simulink model "TEST_TCP"  (R2022b)
settings: Solver=FixedStepAuto  StartTime=0.0  StopTime=inf  FixedStep=1e-3  RelTol=1e-3  EnableMultiTasking=on
undefined symbols (not defined in the file or in its folder): angular, CIRCUIT, CLTF_DAMP, CLTF_FREQ, CLTF_GAIN, CONTROL, CONTROL_INI, DiscIntNeverNeededParam, INPUT, linear, MCP3201, MD25, MODEL, MODEL_INI, mpcstate, MPU60X0, MPU9250, MSG, NAV_MPC_CONTROL, OUTPUT, RCRX, SAMPLING_TIME, SYSID_INPUT, VL6180X
libraries: raspberrypiCommlib x156, simulink x86, dspsigattribs x14, raspberrypiNetworklib x13, embedlinuxBasiclib x9, ctrlSharedLib x2, ros2lib x2, mpclib x1, vrlib x1, sldrtlib x1
(part 17 of 17)

== matlab function TEST_TCP/CONTROL/LOCAL TARGETS/NAVIGATION TARGETS/TRAJECTORY PLANNER (POLYNOMIAL IN Vx & Vy) ==
  data: CONTROL_IN input Bus: CONTROL_Bus; CONTROL output Bus: CONTROL_Bus
function CONTROL = MPC_TARGET_UPDATE(CONTROL_IN)

%--------------------------------------------------------------
% COPY CONTROL BUS
%--------------------------------------------------------------
CONTROL = CONTROL_IN;

%--------------------------------------------------------------
% DISABLING TARGET UPDATE
%--------------------------------------------------------------
% CONTROL_STATUS
% / 0. INITIALIZATION     / 1. ESTIMATION    / 2. ACTIVE CONTROL
if CONTROL.STATE.CONTROL_STATUS < 2  % INITIALIZATION    
    return
end

%--------------------------------------------------------------
% TIME MANAGEMENT
%--------------------------------------------------------------
% Sampling time 
ts = CONTROL.PARAM.SAMPLING_TIME;
% Trajectory update time 
tc = 10*ts;
persistent initialize TIMER
if isempty(initialize)
    TIMER = 0;
    initialize = 1;
end
TIMER = TIMER + ts;
if TIMER > tc-ts/2
    TIMER = 0;
    return
end

%--------------------------------------------------------------
% PARAMETERS
%--------------------------------------------------------------
% Maximun velocity magnitude 
VEL_MAG_MAX = CONTROL.PARAM.VEL_MAG_MAX;
% Prediction horizon (<= prediction horizon in mpcDesigner)
P = 20;
% Circular outline radius
% WP_R = CONTROL.PARAM.WP_R;

%--------------------------------------------------------------
% MEASUREMENTS AND STATE
%--------------------------------------------------------------
VEL_MAG = CONTROL.INPUT.FORWARD_VEL;
VEL_ANG = CONTROL.INPUT.YAW_ANG;
VEL_X = CONTROL.INPUT.EARTH_VEL(1);
VEL_Y = CONTROL.INPUT.EARTH_VEL(2);
POS_XY = CONTROL.INPUT.EARTH_POS(1:2);
WP_XY = CONTROL.TARGET.MISSION_WAYPOINTS(1:CONTROL.TARGET.MISSION_NUM_WAYPOINTS,2:3)';
NEXT_WP = CONTROL.TARGET.MISSION_COUNT;
M = CONTROL.PARAM.NAV_MPC.PRED_HRZ;
if NEXT_WP == size(WP_XY,2)
    CONTROL.TARGET.NAV_REF_LC(1) = 0;
    CONTROL.TARGET.NAV_REF(1) = 0;
    CONTROL.TARGET.NAV_REF_MPC(1:M,1) = zeros(M,1);
    CONTROL.TARGET.VEL_XY_REF(1) = 0;
    CONTROL.TARGET.VEL_XY_REF(2) = 0;
    CONTROL.TARGET.FORWARD_VEL_REF = 0;
end

%--------------------------------------------------------------
% TRAJECTORY PLANNING
%--------------------------------------------------------------
% x(t) = sum(ai*t^i) i=0...N
% y(t) = sum(bi*t^i) i=0...N
% dx(t)/dt = vx(t) = sum(i*ai*t^(i-1)) i=0...N
% dy(t)/dt = vy(t) = sum(i*bi*t^(i-1)) i=0...N
% Position and distance data
pos_x = [POS_XY(1) WP_XY(1,NEXT_WP:end)]';
pos_y = [POS_XY(2) WP_XY(2,NEXT_WP:end)]'; 
d = abs(diff(pos_x) + 1j*diff(pos_y));
% Delete duplicated points (distance = 0)
ind = find(d>0);
pos_x = [pos_x(ind) ; pos_x(end)];
pos_y = [pos_y(ind) ; pos_y(end)];
d = abs(diff(pos_x) + 1j*diff(pos_y));
% Polynomial parameters
Np = min([4 length(pos_x)+1]);
% Polynomial order
N = Np-1;
% Parameter initialization
a = zeros(Np,1);
b = zeros(Np,1);
a(1) = pos_x(1);
b(1) = pos_y(1);
a(2) = VEL_X;
b(2) = VEL_Y;
% Time vector for target
t_tgt = (1:P)'*tc;
VEL_MAG_TARGET = zeros(P,1);
VEL_ANG_TARGET = zeros(P,1);
% Time matrix for velocity target computation
matTp = zeros(P,N+1);
matTv = zeros(P,N);
for nn = 1:N+1
    matTp(:,nn) = t_tgt.^(nn-1);
end
for nn = 1:N
    matTv(:,nn) = nn*t_tgt.^(nn-1);
end
flag_vel_max = true;
k = 1;
while flag_vel_max
    % Reaching time for the next waypoints
    t = cumsum([0 ; k*sqrt(2)*d(1:N-1)/VEL_MAG_MAX]);    
    % Polynomial coefficient estimation 
    % matBx = matA*a(3:Np);  
    % matBy = matA*b(3:Np)
    matA = zeros(Np-2);
    for nn = 1:Np-2
        matA(:,nn) = t(2:end).^(nn+1);
    end
    matBx = pos_x(2:Np-1) - a(2)*t(2:end) - a(1);
    matBy = pos_y(2:Np-1) - b(2)*t(2:end) - b(1);
    inv_matA = inv(matA);
    a(3:end) = inv_matA*matBx;
    b(3:end) = inv_matA*matBy;
    % Position target calculation
    px_tgt = matTp*a;
    py_tgt = matTp*b; 
    % Magnitude and angle velocity targets calculation
    vx_tgt = matTv*a(2:end);
    vy_tgt = matTv*b(2:end); 
    v_tgt = vx_tgt + 1j*vy_tgt;
    VEL_MAG_TARGET = abs(v_tgt);
    VEL_ANG_TARGET = angle(v_tgt)*(VEL_MAG_TARGET(1)>=0.005) + ...
                    VEL_ANG*ones(size(VEL_ANG_TARGET))*(VEL_MAG_TARGET(1)<0.005);
    % Decreasing velocity factor
    k = k*max(VEL_MAG_TARGET)/VEL_MAG_MAX;
    % Maximun velocity verification
    if (max(VEL_MAG_TARGET)/VEL_MAG_MAX)<=1.01
        flag_vel_max = false;
    end
end

%--------------------------------------------------------------
% UNWRAPPING
%--------------------------------------------------------------
aux1 = VEL_ANG_TARGET(1);
aux2 = VEL_ANG;
INC_VEL_ANG_TARGET = zeros(21,1);
INC_VEL_ANG_TARGET(1) = aux1-aux2;
for nn=1:10
    INC_VEL_ANG_TARGET(2*nn:2*nn+1) = [aux1-aux2-2*nn*pi ; aux1-aux2+2*nn*pi];
end
[~,ind] = min(abs(INC_VEL_ANG_TARGET));
VEL_ANG_TARGET(1) = aux2 + INC_VEL_ANG_TARGET(ind);
for nn = 2:P
    INC_VEL_ANG_TARGET = [VEL_ANG_TARGET(nn)-VEL_ANG_TARGET(nn-1)
                          VEL_ANG_TARGET(nn)-VEL_ANG_TARGET(nn-1)-2*pi
                          VEL_ANG_TARGET(nn)-VEL_ANG_TARGET(nn-1)+2*pi];
    [~,ind] = min(abs(INC_VEL_ANG_TARGET));
    VEL_ANG_TARGET(nn) = VEL_ANG_TARGET(nn-1) + INC_VEL_ANG_TARGET(ind);
end

%--------------------------------------------------------------
% CONTROL BUS UPDATE
%--------------------------------------------------------------
CONTROL.TARGET.NAV_REF_LC(1) = VEL_MAG_TARGET(1);
CONTROL.TARGET.NAV_REF_LC(2) = VEL_ANG_TARGET(1);
if M<=P
    CONTROL.TARGET.NAV_REF_MPC(1:M,1) = VEL_MAG_TARGET(1:M);
    CONTROL.TARGET.NAV_REF_MPC(1:M,2) = VEL_ANG_TARGET(1:M);
else
    CONTROL.TARGET.NAV_REF_MPC(1:M,1) = [VEL_MAG_TARGET(1:P); VEL_MAG_TARGET(end)*ones(M-P,1)];
    CONTROL.TARGET.NAV_REF_MPC(1:M,2) = [VEL_ANG_TARGET(1:P); VEL_ANG_TARGET(end)*ones(M-P,1)];
end
VEL_XY = VEL_MAG_TARGET.*exp(1j*VEL_ANG_TARGET);
CONTROL.TARGET.VEL_XY_REF(1) = real(VEL_XY(1));
CONTROL.TARGET.VEL_XY_REF(2) = imag(VEL_XY(1));
CONTROL.TARGET.NAV_REF = [VEL_MAG_TARGET(1) ; VEL_ANG_TARGET(1)];

return

== matlab function TEST_TCP/CONTROL/CONTROL UPDATE  ==
  data: CONTROL_IN input Bus: CONTROL_Bus; CONTROL output Bus: CONTROL_Bus; MOTOR_VOLT output size=2; MOTOR_VOLT_CD output size=2
function [CONTROL,MOTOR_VOLT,MOTOR_VOLT_CD] = CONTROL_UPDATE(CONTROL_IN)

%--------------------------------------------------------------
% COPY CONTROL BUS
%--------------------------------------------------------------
CONTROL = CONTROL_IN;

%--------------------------------------------------------------
% TIMER FOR DIGITAL CONTROL SAMPLING TIME
%--------------------------------------------------------------
persistent TIMER init_1
if isempty(init_1)
    TIMER = 0;
    init_1 = 1;
end
TIMER = TIMER + CONTROL.PARAM.SAMPLING_TIME;

%--------------------------------------------------------------
% CONTROL STATUS
%--------------------------------------------------------------
% / 0. INITIALIZATION     / 1. ESTIMATION    / 2. ACTIVE CONTROL
CONTROL_STATUS = CONTROL.STATE.CONTROL_STATUS;
NUM_DLYS = uint8(floor(CONTROL.PARAM.MOTOR_DELAY/CONTROL.PARAM.CONTROL_SAMPLING_TIME));
if CONTROL_STATUS == 0 || CONTROL_STATUS == 1  % INITIALIZATION OR ESTIMATION
    MOTOR_VOLT = zeros(2,1);
    MOTOR_VOLT_CD = zeros(2,1);
    return
end 

%--------------------------------------------------------------
% DIGITAL CONTROL SAMPLING TIME MANAGEMENT
%--------------------------------------------------------------
if TIMER < CONTROL.PARAM.CONTROL_SAMPLING_TIME
    MOTOR_VOLT = CONTROL.OUTPUT.MOTOR_VOLT;
    MOTOR_VOLT_CD = CONTROL.OUTPUT.MOTOR_VOLT_CD;
    return
else
    TIMER = 0;
end

%--------------------------------------------------------------
% CONTROL MODE
%--------------------------------------------------------------
% / 0. OPEN LOOP / 1. ATTITUDE / 2. VELOCITY / 3. NAVIGATION / 
% / 4. WALL FOLLOWER / 5. WALL-FOLLOWER COMPETITION / 
% / 6. NAVIGATION COMPETITION / 7.FORWARD VELOCITY COMPETITION
CONTROL_MODE = CONTROL.STATE.CONTROL_MODE;
%--------------------------------------------------------------
% VEHICLE MODE
%--------------------------------------------------------------
% / 0. CAR / 1. SELF-BALANCING VEHICLE
VEHICLE_MODE = CONTROL.STATE.VEHICLE_MODE;

%--------------------------------------------------------------
% CONTROL STATE
%--------------------------------------------------------------
persistent init_2 PA_REF_PRV PA_MO_PRV PA_MV_PRV PA_MOD_PRV ...
                      PA_INT_PID_PRV PA_DER_PID_PRV ...
                      YA_REF_PRV YA_MO_PRV YA_MV_PRV YA_MOD_PRV ...
                      YA_INT_PID_PRV YA_DER_PID_PRV ...
                      YR_REF_PRV YR_MO_PRV YR_MV_PRV ...
                      YR_INT_PID_PRV YR_DER_PID_PRV  ...
                      FV_REF_PRV FV_MO_PRV FV_MV_PRV ...
                      FV_INT_PID_PRV FV_DER_PID_PRV  ...
                      WFL_REF_PRV WFL_MO_PRV WFL_MV_PRV ...
                      WFL_INT_PID_PRV WFL_DER_PID_PRV ...
                      SFC_REF_PRV SFC_MO_PRV SFC_MV_PRV ...
                      SFC_STATE_PRV SFC_STATE_INT_PRV  ...
                      NAV_STATE_PRV NAV_STATE_INT_PRV NAV_MV_PRV ...
                      NAV_MO_PRV NAV_REF_PRV ...
                      VEL_SP_STATE YAW_RATE_SP_STATE ...
                      FV_DB_ERR_PRV YR_DB_ERR_PRV FV_DB_MV_PRV YR_DB_MV_PRV ...
                      MAT_NAV_LQR_GS
                                       
% Size of vector and matrices
% Initialization
if isempty(init_2) || CONTROL.STATE.CURRENT_STATUS_SYS==11 % STOP
    PA_REF_PRV = 0;
    PA_MO_PRV = 0;
    PA_MV_PRV = 0;
    PA_MOD_PRV = 0;
    PA_INT_PID_PRV = 0;
    PA_DER_PID_PRV = 0;
    YA_REF_PRV = 0;
    YA_MO_PRV = 0;
    YA_MV_PRV = 0;
    YA_MOD_PRV = 0;
    YA_INT_PID_PRV = 0;
    YA_DER_PID_PRV = 0;
    YR_REF_PRV = 0;
    YR_MO_PRV = 0;
    YR_MV_PRV = 0;
    YR_INT_PID_PRV = 0;
    YR_DER_PID_PRV = 0;
    FV_REF_PRV = 0;
    FV_MO_PRV = 0;
    FV_MV_PRV = 0;
    FV_INT_PID_PRV = 0;
    FV_DER_PID_PRV = 0;
    WFL_REF_PRV = 0.1;
    WFL_MO_PRV = 0.1; 
    WFL_MV_PRV = 0;
    WFL_INT_PID_PRV = 0;
    WFL_DER_PID_PRV = 0;
    SFC_REF_PRV = zeros(2,1);
    SFC_MO_PRV = zeros(2,1);
    SFC_MV_PRV = zeros(2,2);
    SFC_STATE_INT_PRV = zeros(2,1);       
    SFC_STATE_PRV = zeros(6,1);
    SFC_STATE_PRV(4) = CONTROL.INPUT.WALL_DIST; 
    VEL_SP_STATE = zeros(NUM_DLYS+2,1);
    NAV_MV_PRV = zeros(2,2);       
    NAV_STATE_PRV = zeros(6,1);
    NAV_STATE_INT_PRV = zeros(2,1);
    NAV_MO_PRV = zeros(2,1);
    NAV_REF_PRV = zeros(2,1);
    YAW_RATE_SP_STATE = zeros(NUM_DLYS+2,1);
    FV_DB_ERR_PRV = zeros(1,2);
    YR_DB_ERR_PRV = zeros(1,2);
    FV_DB_MV_PRV = zeros(1,2);
    YR_DB_MV_PRV = zeros(1,2);  
    N_calphao = length(CONTROL.PARAM.NAV_SFC.COS_ANG);
    N_vo = length(CONTROL.PARAM.NAV_SFC.FV);
    N_invro = length(CONTROL.PARAM.NAV_SFC.INV_DIST);
    MAT_NAV_LQR_GS = zeros(N_calphao*N_vo*N_invro,3);
    calphao = CONTROL.PARAM.NAV_SFC.COS_ANG;
    vo = CONTROL.PARAM.NAV_SFC.FV;
    invro = CONTROL.PARAM.NAV_SFC.INV_DIST;
    nn = 0;
    for ii = 1:N_calphao
        for jj = 1:N_vo
            for kk = 1:N_invro
                nn = nn + 1;
                MAT_NAV_LQR_GS(nn,:) = [calphao(ii) vo(jj) invro(kk)];
            end
        end
    end
    init_2 = 1;
end

%--------------------------------------------------------------
% INITIALIZATION
%--------------------------------------------------------------
MOTOR_VOLT_CD = zeros(2,1);
NAV_TARGET_REACHED = false;

%-------------------------------------------------------------------------
% ADAPTIVE CONTROL: GAIN SCHEDULING
%-------------------------------------------------------------------------
if CONTROL.STATE.GAIN_SCHEDULING
    % Filtered scheduling variable
    SCHED_VAR = CONTROL.TARGET.FORWARD_VEL_REF;
    % Scheduling variables at operating points
    SCHED_OP = CONTROL.PARAM.OP_STATE(1,:);
    [~,NUM_OP] = min(abs(SCHED_OP-SCHED_VAR));
else
    NUM_OP = double(CONTROL.STATE.FORWARD_VEL_MAIN_OP);
end

%-------------------------------------------------------------------------
% NAVIGATION: ADAPTIVE LQR CONTROL (GAIN SCHEDULING)
%-------------------------------------------------------------------------
if (CONTROL_MODE==3 || CONTROL_MODE==6) && VEHICLE_MODE==0 && ...
              CONTROL.STATE.NAV_CONTROL_TYPE==0
    % OUTPUT COMPUTATION IN POLAR COORDINATES
    NAV_MO_XY = CONTROL.TARGET.NAV_REF - CONTROL.INPUT.NAV_MO;
    NAV_MO_MAG = norm(NAV_MO_XY); % r
    if CONTROL.STATE.NAV_TARGET_REACHED==0
        aux1 = atan2(NAV_MO_XY(2),NAV_MO_XY(1));
        aux2 = CONTROL.TARGET.YAW_ANG_REF;
        INC_ANG = zeros(41,1);
        INC_ANG(1) = aux1-aux2;
        for ii = 1:20
            INC_ANG(2*ii)   = aux1-aux2-2*ii*pi;
            INC_ANG(2*ii+1) = aux1-aux2+2*ii*pi;
        end
        [~,ind] = min(abs(INC_ANG));
        CONTROL.TARGET.YAW_ANG_REF = aux2 + INC_ANG(ind); % phi
    end
    NAV_MO_ANG = CONTROL.TARGET.YAW_ANG_REF - CONTROL.INPUT.YAW_ANG; % alpha = phi - shi
    if abs(NAV_MO_MAG)>CONTROL.PARAM.NAV_MAX_TARGET_RADIUS
        NAV_MO_MAG = CONTROL.PARAM.NAV_MAX_TARGET_RADIUS; % r
    end
    NAV_STATE = [CONTROL.INPUT.FORWARD_VEL ; CONTROL.INPUT.YAW_RATE ; ...
                 CONTROL.INPUT.FV_INT_ERROR ; CONTROL.INPUT.YR_INT_ERROR ; ...
                 NAV_MO_MAG ; NAV_MO_ANG];
    if NAV_MO_MAG<=CONTROL.PARAM.NAV_STOP_RADIUS
       NAV_MO_MAG = 0; % r = 0
       NAV_MO_ANG = 0; % alpha = 0;
       NAV_STATE = zeros(6,1);
       NAV_STATE_PRV = zeros(6,1);
       NAV_STATE_INT_PRV = zeros(2,1);
       NAV_MO_PRV = zeros(2,1);
       NAV_REF_PRV = zeros(2,1);
       CONTROL.STATE.NAV_TARGET_REACHED = uint8(1);
    else
        CONTROL.STATE.NAV_TARGET_REACHED = uint8(0);
    end
    NAV_REF = [0 ; 0];
    NAV_MO = [NAV_MO_MAG ; NAV_MO_ANG];
    % GAIN MATRICES TO BE APPLIED
    SANG = sin(NAV_MO_ANG);
    signSANG = SANG>=0;
    CANG = cos(NAV_MO_ANG);
    signCANG = CANG>=0;
    absCANG = abs(CANG);    
    FV = CONTROL.INPUT.FORWARD_VEL;
    INVR = (1/(NAV_MO_MAG+(NAV_MO_MAG<0.01)))*(NAV_MO_MAG>0.01) + 100*(NAV_MO_MAG<=0.01);
    if signCANG && signSANG
        NAV_MATRIX = CONTROL.PARAM.NAV_SFC.KPP;
    elseif signCANG && ~signSANG
        NAV_MATRIX = CONTROL.PARAM.NAV_SFC.KPN;
    elseif ~signCANG && signSANG
        NAV_MATRIX = CONTROL.PARAM.NAV_SFC.KNP;
    else
        NAV_MATRIX = CONTROL.PARAM.NAV_SFC.KNN;
    end
    [~,ind] = min(sum(abs([MAT_NAV_LQR_GS(:,1:2) MAT_NAV_LQR_GS(:,3)/100]-repmat([absCANG FV INVR/100],size(NAV_MATRIX,1),1)),2));
    % INPUTS
    NAV_INPUT.MO_PRV = NAV_MO_PRV;
    NAV_INPUT.REF_PRV = NAV_REF_PRV;
    NAV_INPUT.STATE_PRV = NAV_STATE_PRV;
    NAV_INPUT.STATE = NAV_STATE;
    NAV_INPUT.MV_PRV = NAV_MV_PRV;
    NAV_INPUT.STATE_INT = NAV_STATE_INT_PRV;
    % PARAMETERS
    NAV_PARAM.ts = CONTROL.PARAM.CONTROL_SAMPLING_TIME;
    NAV_PARAM.MV_MAX = CONTROL.PARAM.NAV_MV_MAX;
    NAV_PARAM.MV_MIN = CONTROL.PARAM.NAV_MV_MIN;
    NAV_PARAM.OP_INPUT = zeros(2,1);
    NAV_PARAM.OP_STATE = zeros(6,1);
    NAV_PARAM.OP_OUTPUT = zeros(2,1);
    NAV_PARAM.Kr = zeros(2,2);
    NAV_PARAM.Kd = zeros(2,2);
    NAV_PARAM.K = [NAV_MATRIX(ind,1:6) ; NAV_MATRIX(ind,7:12)];
    NAV_PARAM.Ki = [NAV_MATRIX(ind,13:14) ; NAV_MATRIX(ind,15:16)];
    NAV_PARAM.INT_DISC_TYPE = CONTROL.PARAM.FORWARD_VEL_SFC.INT_DISC_TYPE;
    NAV_PARAM.ANTIWINDUP = uint8(1);
    NAV_INPUT.REF = NAV_REF;
    NAV_INPUT.MO = NAV_MO;
    % STATE-FEEDBACK CONTROL
    NAV_OUTPUT = SFC(NAV_INPUT,NAV_PARAM);
    % OUTPUTS
    NAV_MV_PRV = [NAV_OUTPUT.MV NAV_MV_PRV(:,1:end-1)];
    NAV_REF_PRV = NAV_INPUT.REF;
    NAV_MO_PRV = NAV_INPUT.MO;
    NAV_STATE_PRV = NAV_INPUT.STATE;
    NAV_STATE_INT_PRV = NAV_OUTPUT.STATE_INT; 
    if CONTROL.STATE.NAV_TARGET_REACHED==0
        CONTROL.TARGET.FORWARD_VEL_REF = NAV_OUTPUT.MV(1);
        CONTROL.TARGET.YAW_RATE_REF = NAV_OUTPUT.MV(2);
    else
        CONTROL.TARGET.FORWARD_VEL_REF = 0;
        CONTROL.TARGET.YAW_RATE_REF = 0;
    end
end

%-------------------------------------------------------------------------
% WALL DISTANCE: PID 
%-------------------------------------------------------------------------
if (CONTROL_MODE==4 || CONTROL_MODE==5) && CONTROL.STATE.WFL_CONTROL_TYPE<2  
    % INPUTS
    PID_INPUT.REF = CONTROL.TARGET.WALL_DIST_REF;
    PID_INPUT.REF_PRV = WFL_REF_PRV;
    PID_INPUT.MO = CONTROL.INPUT.WALL_DIST;
    PID_INPUT.MO_PRV = WFL_MO_PRV;
    PID_INPUT.INT_PID_PRV = WFL_INT_PID_PRV;
    PID_INPUT.DER_PID_PRV = WFL_DER_PID_PRV;
    PID_INPUT.MV_PRV = WFL_MV_PRV(1);
    PID_INPUT.MOD = 0;
    PID_INPUT.MOD_PRV = 0;
    PID_INPUT.MV_PID_PRV = 0;
    PID_INPUT.STATE = 0;
    PID_INPUT.STATE_PRV = 0;
    PID_INPUT.STATE_DCP = 0;
    % PARAMETERS
    PID_PARAM.ts = CONTROL.PARAM.CONTROL_SAMPLING_TIME;
    if CONTROL.STATE.WFL_CONTROL_TYPE
        PID_PARAM.K = CONTROL.PARAM.WFL_CD_PID.K(NUM_OP,1);
        PID_PARAM.Ti = CONTROL.PARAM.WFL_CD_PID.Ti(NUM_OP,1);
        PID_PARAM.Td = CONTROL.PARAM.WFL_CD_PID.Td(NUM_OP,1);
        PID_PARAM.b = CONTROL.PARAM.WFL_CD_PID.b(NUM_OP,1);
        PID_PARAM.N = CONTROL.PARAM.WFL_CD_PID.N(NUM_OP,1);
        PID_PARAM.MV_MAX = 1e6;
        PID_PARAM.MV_MIN = -1e6;
        PID_PARAM.INT_DISC_TYPE = CONTROL.PARAM.WFL_CD_PID.INT_DISC_TYPE;
        PID_PARAM.DER_DISC_TYPE = CONTROL.PARAM.WFL_CD_PID.DER_DISC_TYPE;
        PID_PARAM.DER_INPUT = CONTROL.PARAM.WFL_CD_PID.DER_INPUT;
        PID_PARAM.ANTIWINDUP = CONTROL.PARAM.WFL_CD_PID.ANTIWINDUP;
    else
        PID_PARAM.K = CONTROL.PARAM.WFL_SL_PID.K(NUM_OP,1);
        PID_PARAM.Ti = CONTROL.PARAM.WFL_SL_PID.Ti(NUM_OP,1);
        PID_PARAM.Td = CONTROL.PARAM.WFL_SL_PID.Td(NUM_OP,1);
        PID_PARAM.b = CONTROL.PARAM.WFL_SL_PID.b(NUM_OP,1);
        PID_PARAM.N = CONTROL.PARAM.WFL_SL_PID.N(NUM_OP,1);
        PID_PARAM.MV_MAX = 1e6;
        PID_PARAM.MV_MIN = -1e6;
        PID_PARAM.INT_DISC_TYPE = CONTROL.PARAM.WFL_SL_PID.INT_DISC_TYPE;
        PID_PARAM.DER_DISC_TYPE = CONTROL.PARAM.WFL_SL_PID.DER_DISC_TYPE;
        PID_PARAM.DER_INPUT = CONTROL.PARAM.WFL_SL_PID.DER_INPUT;
        PID_PARAM.ANTIWINDUP = CONTROL.PARAM.WFL_SL_PID.ANTIWINDUP;
    end
    % PID CONTROL
    PID_OUTPUT = PID_MV(PID_INPUT,PID_PARAM);
    % OUTPUTS
    WFL_MV_PRV = PID_OUTPUT.MV;
    if CONTROL.STATE.WFL_CONTROL_TYPE
        CONTROL.TARGET.YAW_ANG_REF = PID_OUTPUT.MV;
    else
        MOTOR_VOLT_CD(2) = PID_OUTPUT.MV + ...
            double(CONTROL.STATE.WFL_FEEDFORWARD)*CONTROL.PARAM.MOTOR_VOLT_DROP_DIF;
    end
    WFL_REF_PRV = CONTROL.TARGET.WALL_DIST_REF;
    WFL_MO_PRV = CONTROL.INPUT.WALL_DIST;
    WFL_INT_PID_PRV = PID_OUTPUT.INT;
    WFL_DER_PID_PRV = PID_OUTPUT.DER;
end

%-------------------------------------------------------------------------
% STATE FEEDBACK CONTROL DEFINITION
%-------------------------------------------------------------------------
SFC_PARAM.K = zeros(2,6);
SFC_PARAM.Ki = zeros(2,2);
SFC_PARAM.Kr = zeros(2,2);
SFC_PARAM.Kd = zeros(2,2);
SFC_PARAM.INT_DISC_TYPE = uint8(0);
SFC_PARAM.ANTIWINDUP = uint8(0);
SFC_INPUT.REF = zeros(2,1);
SFC_INPUT.MO = zeros(2,1);
SFC_PARAM.OP_OUTPUT = zeros(2,1);
FLAG_SFC = uint8(0);
FLAG_MV = uint8([0 0]);
% FORWARD VELOCITY AND STATE FEEDBACK CONTROL AND CAR MODE
if CONTROL_MODE>0 && CONTROL_MODE<8 && CONTROL.STATE.FORWARD_VEL_CONTROL_TYPE==1 && VEHICLE_MODE==0
    SFC_PARAM.K(1,1) = CONTROL.PARAM.FORWARD_VEL_SFC.K(1,1);
    SFC_PARAM.Ki(1,1) = CONTROL.PARAM.FORWARD_VEL_SFC.Ki;
    SFC_PARAM.INT_DISC_TYPE = CONTROL.PARAM.FORWARD_VEL_SFC.INT_DISC_TYPE;
    SFC_PARAM.ANTIWINDUP = uint8(1);
    SFC_INPUT.REF(1) = CONTROL.TARGET.FORWARD_VEL_REF;
    SFC_INPUT.MO(1) = CONTROL.INPUT.FORWARD_VEL;
    FLAG_SFC = uint8(1);
    FLAG_MV(1) = uint8(1);
end
% FORWARD VELOCITY AND STATE FEEDBACK CONTROL AND SELF-BALANCING VEHICLE
if CONTROL_MODE>0 && CONTROL_MODE<8 && ...
        CONTROL.STATE.FORWARD_VEL_CONTROL_TYPE==1 && VEHICLE_MODE==1
    SFC_PARAM.K(1,[1 5 6]) = CONTROL.PARAM.FORWARD_VEL_SFC.K;
    SFC_PARAM.Ki(1,1) = CONTROL.PARAM.FORWARD_VEL_SFC.Ki;
    SFC_PARAM.INT_DISC_TYPE = CONTROL.PARAM.FORWARD_VEL_SFC.INT_DISC_TYPE;
    SFC_PARAM.ANTIWINDUP = uint8(1);
    SFC_INPUT.REF(1) = CONTROL.TARGET.FORWARD_VEL_REF;
    SFC_INPUT.MO(1) = CONTROL.INPUT.FORWARD_VEL;
    FLAG_SFC = uint8(1);
    FLAG_MV(1) = uint8(1);
end
% YAW RATE AND STATE FEEDBACK CONTROL
if (CONTROL_MODE==2 || CONTROL_MODE==3 || CONTROL_MODE==6) && ...
        CONTROL.STATE.YAW_RATE_CONTROL_TYPE==1
    SFC_PARAM.K(2,2) = CONTROL.PARAM.YAW_RATE_SFC.K;
    SFC_PARAM.Ki(2,2) = CONTROL.PARAM.YAW_RATE_SFC.Ki;
    SFC_PARAM.INT_DISC_TYPE = CONTROL.PARAM.YAW_RATE_SFC.INT_DISC_TYPE;
    SFC_PARAM.ANTIWINDUP = uint8(1);
    SFC_INPUT.REF(2) = CONTROL.TARGET.YAW_RATE_REF;
    SFC_INPUT.MO(2) = CONTROL.INPUT.YAW_RATE;
    FLAG_SFC = uint8(1);
    FLAG_MV(2) = uint8(1);
end
% YAW ANGLE AND STATE FEEDBACK CONTROL
if (CONTROL_MODE==1) &&  CONTROL.STATE.YAW_ANG_CONTROL_TYPE==1
    SFC_PARAM.K(2,2:3) = CONTROL.PARAM.YAW_ANG_SFC.K;
    SFC_PARAM.Ki(2,2) = CONTROL.PARAM.YAW_ANG_SFC.Ki;
    SFC_PARAM.INT_DISC_TYPE = CONTROL.PARAM.YAW_ANG_SFC.INT_DISC_TYPE;
    SFC_PARAM.ANTIWINDUP = uint8(1);
    SFC_INPUT.REF(2) = CONTROL.TARGET.YAW_ANG_REF;
    SFC_INPUT.MO(2) = CONTROL.INPUT.YAW_ANG;
    FLAG_SFC = uint8(1);
    FLAG_MV(2) = uint8(1);
end
% PITCH ANGLE AND STATE FEEDBACK CONTROL
if CONTROL_MODE==8 && CONTROL.STATE.PITCH_ANG_CONTROL_TYPE>0 && VEHICLE_MODE==1
    if CONTROL.STATE.PITCH_ANG_CONTROL_TYPE==1
        SFC_PARAM.K(1,[1 5 6]) = CONTROL.PARAM.PITCH_ANG_SFC.K;
        SFC_PARAM.Ki(1,1) = 0;
        SFC_PARAM.INT_DISC_TYPE = uint8(0);
        SFC_PARAM.ANTIWINDUP = uint8(0);
        SFC_INPUT.MO(1) = CONTROL.INPUT.PITCH_ANG;
    else
        SFC_PARAM.K(1,[1 5 6]) = CONTROL.PARAM.FORWARD_VEL_SFC.K;
        SFC_PARAM.Ki(1,1) = CONTROL.PARAM.FORWARD_VEL_SFC.Ki;
        SFC_PARAM.INT_DISC_TYPE = CONTROL.PARAM.FORWARD_VEL_SFC.INT_DISC_TYPE;
        SFC_PARAM.ANTIWINDUP = uint8(1);
        SFC_INPUT.REF(1) = 0;
        SFC_INPUT.MO(1) = CONTROL.INPUT.FORWARD_VEL;
    end
    FLAG_SFC = uint8(1);
    FLAG_MV(1) = uint8(1);
end
% WALL FOLLOWER AND STATE FEEDBACK CONTROL
if (CONTROL_MODE==4 || CONTROL_MODE==5) && ...
        CONTROL.STATE.WFL_CONTROL_TYPE>1    
    SFC_PARAM.K(2,2:4) = CONTROL.PARAM.WFL_SFC.K(NUM_OP,:);
    SFC_PARAM.OP_OUTPUT(2) = CONTROL.PARAM.OP_OUTPUT(3,NUM_OP);
    FLAG_SFC = uint8(1);
    FLAG_MV(2) = uint8(1);
end

%-------------------------------------------------------------------------
% STATE-FEEDBACK CONTROL
%-------------------------------------------------------------------------
if FLAG_SFC
    % INPUTS
    SFC_INPUT.MO_PRV = SFC_MO_PRV;
    SFC_INPUT.REF_PRV = SFC_REF_PRV;
    SFC_INPUT.STATE = CONTROL.INPUT.STATE(1:6);
    SFC_INPUT.STATE_PRV = SFC_STATE_PRV;
    SFC_INPUT.MV_PRV = SFC_MV_PRV;
    SFC_INPUT.STATE_INT = SFC_STATE_INT_PRV;
    % PARAMETERS
    SFC_PARAM.ts = CONTROL.PARAM.CONTROL_SAMPLING_TIME;
    SFC_PARAM.MV_MAX = +1e6;
    SFC_PARAM.MV_MIN = -1e6;
    OP_MOTOR_VOLT = CONTROL.PARAM.OP_INPUT(1:2,NUM_OP);
    OP_MOTOR_VOLT_CD = [sum(OP_MOTOR_VOLT) ; -diff(OP_MOTOR_VOLT)]/2;
    SFC_PARAM.OP_INPUT = OP_MOTOR_VOLT_CD;
    % SFC_PARAM.OP_STATE = [CONTROL.PARAM.OP_STATE(:,NUM_OP) ; 0 ; 0]; 
    SFC_PARAM.OP_STATE = [CONTROL.PARAM.OP_STATE(:,NUM_OP)];
    SFC_PARAM.OP_STATE(4) = CONTROL.TARGET.WALL_DIST_REF;
    % STATE-FEEDBACK CONTROL
    SFC_OUTPUT = SFC(SFC_INPUT,SFC_PARAM);
    % OUTPUTS
    SFC_MV_PRV = [SFC_OUTPUT.MV SFC_MV_PRV(:,1:end-1)];
    SFC_REF_PRV = SFC_INPUT.REF;
    SFC_MO_PRV = SFC_INPUT.MO;
    SFC_STATE_PRV = SFC_INPUT.STATE;
    SFC_STATE_INT_PRV = SFC_OUTPUT.STATE_INT; 
    if CONTROL_MODE==2 || CONTROL_MODE==3 || CONTROL_MODE==6 
        % FORWARD-VELOCITY INTEGRAL ERROR
        CONTROL.INPUT.FV_INT_ERROR = SFC_OUTPUT.STATE_INT(1);
        % YAW-RATE INTEGRAL ERROR
        CONTROL.INPUT.YR_INT_ERROR = SFC_OUTPUT.STATE_INT(2);
    end
    if FLAG_MV(1)
        MOTOR_VOLT_CD(1) = SFC_OUTPUT.MV(1);
    end
    if FLAG_MV(2)
        MOTOR_VOLT_CD(2) = SFC_OUTPUT.MV(2) + ...
            double(CONTROL.STATE.WFL_FEEDFORWARD)*CONTROL.PARAM.MOTOR_VOLT_DROP_DIF;
    end
    if (CONTROL_MODE==3 || CONTROL_MODE==6) && CONTROL.STATE.NAV_TARGET_REACHED==1
        MOTOR_VOLT_CD(1) = 0;
        MOTOR_VOLT_CD(2) = 0;
    end
    
end

%-------------------------------------------------------------------------
% FORWARD VELOCITY: PID CONTROL
%-------------------------------------------------------------------------
if CONTROL_MODE>0 && CONTROL_MODE<8 && CONTROL.STATE.FORWARD_VEL_CONTROL_TYPE==0  
    % SMITH PREDICTOR
    if CONTROL.STATE.SP_MODE(1)==1 && VEHICLE_MODE==0
        % PARAMETERS
        SCALE_FACTOR = 0.5;
        if NUM_DLYS==1
            SCALE_FACTOR = 0.25;
        end
        Km = CONTROL.PARAM.VEL_GAIN;
        Tm = CONTROL.PARAM.VEL_TIME_CONSTANT;
        if CONTROL.STATE.OBSERVER_MODE== 1 % EKF
            Tf = 1/2/pi/CONTROL.PARAM.EKF_FILT_FREQ;   
        else
            Tf = 1/2/pi/CONTROL.PARAM.ENC_FILT_FREQ;   
        end
        % PLANT DISCRETIZATION
        p1 = exp(-CONTROL.PARAM.CONTROL_SAMPLING_TIME/Tm);
        p2 = exp(-CONTROL.PARAM.CONTROL_SAMPLING_TIME/Tf);
        R1 = Tm/(Tf-Tm);
        R2 = Tf/(Tm-Tf);
        B1 = -Km*(p1+p2+R1*(1+p2)+R2*(1+p1));
        B0 = Km*(p1*p2+R1*p2+R2*p1);
        A1 = -(p1+p2);
        A0 = p1*p2;
        % COMPENSATOR DESIGN
        matAd = [-A1 -A0 zeros(1,NUM_DLYS) ; eye(NUM_DLYS+1) zeros(NUM_DLYS+1,1)];
        matBd = [SCALE_FACTOR ; zeros(NUM_DLYS+1,1)];
        matCd = [B1 B0 zeros(1,NUM_DLYS-2) -B1 -B0]/SCALE_FACTOR;
        if NUM_DLYS==1
            matCd = [B1 -B1+B0 -B0]/SCALE_FACTOR;
        end
        matDd = 0;
        % INPUT
        % VEL_SP_INPUT = CONTROL.OUTPUT.MOTOR_VOLT_CD(1);
        VEL_SP_INPUT = FV_MV_PRV(1);
        % STATE-SPACE UPDATE
        AUX = matAd*VEL_SP_STATE + matBd*VEL_SP_INPUT;
        VEL_SP_STATE = AUX(1:length(VEL_SP_STATE));
        VEL_SP_OUTPUT = matCd*VEL_SP_STATE + matDd*VEL_SP_INPUT;
    else
        VEL_SP_OUTPUT = 0;
    end 
    % INPUTS
    PID_INPUT.REF = CONTROL.TARGET.FORWARD_VEL_REF;
    PID_INPUT.REF_PRV = FV_REF_PRV;
    PID_INPUT.MO = CONTROL.INPUT.FORWARD_VEL + VEL_SP_OUTPUT;
    PID_INPUT.MO_PRV = FV_MO_PRV;
    PID_INPUT.INT_PID_PRV = FV_INT_PID_PRV;
    PID_INPUT.DER_PID_PRV = FV_DER_PID_PRV;
    PID_INPUT.MV_PRV = FV_MV_PRV(1);
    PID_INPUT.MOD = 0;
    PID_INPUT.MOD_PRV = 0;
    PID_INPUT.MV_PID_PRV = 0;
    PID_INPUT.STATE = 0;
    PID_INPUT.STATE_PRV = 0;
    PID_INPUT.STATE_DCP = 0;
    % PARAMETERS
    PID_PARAM.ts = CONTROL.PARAM.CONTROL_SAMPLING_TIME;
    PID_PARAM.K = CONTROL.PARAM.FORWARD_VEL_PID.K;
    PID_PARAM.Ti = CONTROL.PARAM.FORWARD_VEL_PID.Ti;
    PID_PARAM.Td = CONTROL.PARAM.FORWARD_VEL_PID.Td;
    PID_PARAM.b = CONTROL.PARAM.FORWARD_VEL_PID.b;
    PID_PARAM.N = CONTROL.PARAM.FORWARD_VEL_PID.N;
    PID_PARAM.MV_MAX = 1e6;
    PID_PARAM.MV_MIN = -1e6;
    PID_PARAM.INT_DISC_TYPE = CONTROL.PARAM.FORWARD_VEL_PID.INT_DISC_TYPE;
    PID_PARAM.DER_DISC_TYPE = CONTROL.PARAM.FORWARD_VEL_PID.DER_DISC_TYPE;
    PID_PARAM.DER_INPUT = CONTROL.PARAM.FORWARD_VEL_PID.DER_INPUT;
    PID_PARAM.ANTIWINDUP = CONTROL.PARAM.FORWARD_VEL_PID.ANTIWINDUP;
    % PID CONTROL
    PID_OUTPUT = PID_MV(PID_INPUT,PID_PARAM);
    % OUTPUTS
    FV_MV_PRV = [PID_OUTPUT.MV FV_MV_PRV(1:end-1)];
    if VEHICLE_MODE == 0
        MOTOR_VOLT_CD(1) = PID_OUTPUT.MV;
    else
        CONTROL.TARGET.PITCH_ANG_REF = PID_OUTPUT.MV;
    end
    FV_REF_PRV = CONTROL.TARGET.FORWARD_VEL_REF;
    FV_MO_PRV = CONTROL.INPUT.FORWARD_VEL + VEL_SP_OUTPUT;
    FV_INT_PID_PRV = PID_OUTPUT.INT;
    FV_DER_PID_PRV = PID_OUTPUT.DER;
end

%-------------------------------------------------------------------------
% YAW RATE: PID CONTROL
%-------------------------------------------------------------------------
if (CONTROL_MODE==2 || CONTROL_MODE==7) && CONTROL.STATE.YAW_RATE_CONTROL_TYPE==0  
    if CONTROL.STATE.SP_MODE(2)==1 && VEHICLE_MODE==0
        % PARAMETERS
        SCALE_FACTOR = 0.5;
        if NUM_DLYS==1
            SCALE_FACTOR = 0.25;
        end
        Km = CONTROL.PARAM.YAW_RATE_GAIN;
        Tm = CONTROL.PARAM.YAW_RATE_TIME_CONSTANT;
        if CONTROL.STATE.OBSERVER_MODE== 1 % EKF
            Tf = 1/2/pi/CONTROL.PARAM.EKF_FILT_FREQ;   
        else
            Tf = 1/2/pi/CONTROL.PARAM.ENC_FILT_FREQ;   
        end
        % PLANT DISCRETIZATION
        p1 = exp(-CONTROL.PARAM.CONTROL_SAMPLING_TIME/Tm);
        p2 = exp(-CONTROL.PARAM.CONTROL_SAMPLING_TIME/Tf);
        R1 = Tm/(Tf-Tm);
        R2 = Tf/(Tm-Tf);
        B1 = -Km*(p1+p2+R1*(1+p2)+R2*(1+p1));
        B0 = Km*(p1*p2+R1*p2+R2*p1);
        A1 = -(p1+p2);
        A0 = p1*p2;
        % COMPENSATOR DESIGN
        matAd = [-A1 -A0 zeros(1,NUM_DLYS) ; eye(NUM_DLYS+1) zeros(NUM_DLYS+1,1)];
        matBd = [SCALE_FACTOR ; zeros(NUM_DLYS+1,1)];
        matCd = [B1 B0 zeros(1,NUM_DLYS-2) -B1 -B0]/SCALE_FACTOR;
        if NUM_DLYS==1
            matCd = [B1 -B1+B0 -B0]/SCALE_FACTOR;
        end
        matDd = 0;
        % INPUT
        % YAW_RATE_SP_INPUT = CONTROL.OUTPUT.MOTOR_VOLT_CD(2);
        YAW_RATE_SP_INPUT = YR_MV_PRV(1);
        % STATE-SPACE UPDATE
        AUX = matAd*YAW_RATE_SP_STATE + matBd*YAW_RATE_SP_INPUT;
        YAW_RATE_SP_STATE = AUX(1:length(YAW_RATE_SP_STATE));
        YAW_RATE_SP_OUTPUT = matCd*YAW_RATE_SP_STATE + matDd*YAW_RATE_SP_INPUT;
    else
        YAW_RATE_SP_OUTPUT = 0;
    end
    % INPUTS
    PID_INPUT.REF = CONTROL.TARGET.YAW_RATE_REF;
    PID_INPUT.REF_PRV = YR_REF_PRV;
    PID_INPUT.MO = CONTROL.INPUT.YAW_RATE + YAW_RATE_SP_OUTPUT;
    PID_INPUT.MO_PRV = YR_MO_PRV;
    PID_INPUT.INT_PID_PRV = YR_INT_PID_PRV;
    PID_INPUT.DER_PID_PRV = YR_DER_PID_PRV;
    PID_INPUT.MV_PRV = YR_MV_PRV(1);
    PID_INPUT.MOD = 0;
    PID_INPUT.MOD_PRV = 0;
    PID_INPUT.MV_PID_PRV = 0;
    PID_INPUT.STATE = 0;
    PID_INPUT.STATE_PRV = 0;
    PID_INPUT.STATE_DCP = 0;
    % PARAMETERS
    PID_PARAM.ts = CONTROL.PARAM.CONTROL_SAMPLING_TIME;
    PID_PARAM.K = CONTROL.PARAM.YAW_RATE_PID.K;
    PID_PARAM.Ti = CONTROL.PARAM.YAW_RATE_PID.Ti;
    PID_PARAM.Td = CONTROL.PARAM.YAW_RATE_PID.Td;
    PID_PARAM.b = CONTROL.PARAM.YAW_RATE_PID.b;
    PID_PARAM.N = CONTROL.PARAM.YAW_RATE_PID.N;
    PID_PARAM.MV_MAX = 1e6;
    PID_PARAM.MV_MIN = -1e6;
    PID_PARAM.INT_DISC_TYPE = CONTROL.PARAM.YAW_RATE_PID.INT_DISC_TYPE;
    PID_PARAM.DER_DISC_TYPE = CONTROL.PARAM.YAW_RATE_PID.DER_DISC_TYPE;
    PID_PARAM.DER_INPUT = CONTROL.PARAM.YAW_RATE_PID.DER_INPUT;
    PID_PARAM.ANTIWINDUP = CONTROL.PARAM.YAW_RATE_PID.ANTIWINDUP;
    % PID CONTROL
    PID_OUTPUT = PID_MV(PID_INPUT,PID_PARAM);
    % OUTPUTS
    YR_MV_PRV = [PID_OUTPUT.MV YR_MV_PRV(1:end-1)];
    % MOTOR_VOLT_CD(2) = PID_OUTPUT.MV;
    MOTOR_VOLT_CD(2) = PID_OUTPUT.MV + ...
            double(CONTROL.STATE.WFL_FEEDFORWARD)*CONTROL.PARAM.MOTOR_VOLT_DROP_DIF;
    YR_REF_PRV = CONTROL.TARGET.YAW_RATE_REF;
    YR_MO_PRV = CONTROL.INPUT.YAW_RATE + YAW_RATE_SP_OUTPUT;
    YR_INT_PID_PRV = PID_OUTPUT.INT;
    YR_DER_PID_PRV = PID_OUTPUT.DER;
end

%-------------------------------------------------------------------------
% YAW ANGLE: PID CONTROL
%-------------------------------------------------------------------------
if ((CONTROL_MODE==4 || CONTROL_MODE==5) && CONTROL.STATE.WFL_CONTROL_TYPE==1) || ...
   (CONTROL_MODE==1 && CONTROL.STATE.YAW_ANG_CONTROL_TYPE==0)        
    % INPUTS
    PID_INPUT.REF = CONTROL.TARGET.YAW_ANG_REF;
    PID_INPUT.REF_PRV = YA_REF_PRV;
    PID_INPUT.MO = CONTROL.INPUT.YAW_ANG;
    PID_INPUT.MO_PRV = YA_MO_PRV;
    PID_INPUT.INT_PID_PRV = YA_INT_PID_PRV;
    PID_INPUT.DER_PID_PRV = YA_DER_PID_PRV;
    PID_INPUT.MV_PRV = YA_MV_PRV(1);
    PID_INPUT.MOD = CONTROL.INPUT.YAW_RATE;
    PID_INPUT.MOD_PRV = YA_MOD_PRV;
    PID_INPUT.MV_PID_PRV = 0;
    PID_INPUT.STATE = 0;
    PID_INPUT.STATE_PRV = 0;
    PID_INPUT.STATE_DCP = 0;
    % PARAMETERS
    PID_PARAM.ts = CONTROL.PARAM.CONTROL_SAMPLING_TIME;
    PID_PARAM.K = CONTROL.PARAM.YAW_ANG_PID.K;
    PID_PARAM.Ti = CONTROL.PARAM.YAW_ANG_PID.Ti;
    PID_PARAM.Td = CONTROL.PARAM.YAW_ANG_PID.Td;
    PID_PARAM.b = CONTROL.PARAM.YAW_ANG_PID.b;
    PID_PARAM.N = CONTROL.PARAM.YAW_ANG_PID.N;
    PID_PARAM.MV_MAX = 1e6;
    PID_PARAM.MV_MIN = -1e6;
    PID_PARAM.INT_DISC_TYPE = CONTROL.PARAM.YAW_ANG_PID.INT_DISC_TYPE;
    PID_PARAM.DER_DISC_TYPE = CONTROL.PARAM.YAW_ANG_PID.DER_DISC_TYPE;
    PID_PARAM.DER_INPUT = CONTROL.PARAM.YAW_ANG_PID.DER_INPUT;
    PID_PARAM.ANTIWINDUP = CONTROL.PARAM.YAW_ANG_PID.ANTIWINDUP;
    % PID CONTROL
    PID_OUTPUT = PID_MV(PID_INPUT,PID_PARAM);
    % OUTPUTS
    YA_MV_PRV = [PID_OUTPUT.MV YA_MV_PRV(1:end-1)];
    MOTOR_VOLT_CD(2) = PID_OUTPUT.MV + ...
            double(CONTROL.STATE.WFL_FEEDFORWARD)*CONTROL.PARAM.MOTOR_VOLT_DROP_DIF;
    YA_REF_PRV = CONTROL.TARGET.YAW_ANG_REF;
    YA_MO_PRV = CONTROL.INPUT.YAW_ANG;
    YA_MOD_PRV = CONTROL.INPUT.YAW_RATE;
    YA_INT_PID_PRV = PID_OUTPUT.INT;
    YA_DER_PID_PRV = PID_OUTPUT.DER;
end

%-------------------------------------------------------------------------
% PITCH ANGLE: PID CONTROL
%-------------------------------------------------------------------------
if ((CONTROL_MODE>0 && CONTROL_MODE<8 && CONTROL.STATE.FORWARD_VEL_CONTROL_TYPE==0) || ...
   (CONTROL_MODE==8 && CONTROL.STATE.PITCH_ANG_CONTROL_TYPE==0)) && ...
   VEHICLE_MODE==1        
    % INPUTS
    PID_INPUT.REF = CONTROL.TARGET.PITCH_ANG_REF;
    PID_INPUT.REF_PRV = PA_REF_PRV;
    PID_INPUT.MO = CONTROL.INPUT.PITCH_ANG;
    PID_INPUT.MO_PRV = PA_MO_PRV;
    PID_INPUT.INT_PID_PRV = PA_INT_PID_PRV;
    PID_INPUT.DER_PID_PRV = PA_DER_PID_PRV;
    PID_INPUT.MV_PRV = PA_MV_PRV(1);
    PID_INPUT.MOD = CONTROL.INPUT.PITCH_RATE;
    PID_INPUT.MOD_PRV = PA_MOD_PRV;
    PID_INPUT.MV_PID_PRV = 0;
    PID_INPUT.STATE = 0;
    PID_INPUT.STATE_PRV = 0;
    PID_INPUT.STATE_DCP = 0;
    % PARAMETERS
    PID_PARAM.ts = CONTROL.PARAM.CONTROL_SAMPLING_TIME;
    PID_PARAM.K = CONTROL.PARAM.PITCH_ANG_PID.K;
    PID_PARAM.Ti = CONTROL.PARAM.PITCH_ANG_PID.Ti;
    PID_PARAM.Td = CONTROL.PARAM.PITCH_ANG_PID.Td;
    PID_PARAM.b = CONTROL.PARAM.PITCH_ANG_PID.b;
    PID_PARAM.N = CONTROL.PARAM.PITCH_ANG_PID.N;
    PID_PARAM.MV_MAX = 1e6;
    PID_PARAM.MV_MIN = -1e6;
    PID_PARAM.INT_DISC_TYPE = CONTROL.PARAM.PITCH_ANG_PID.INT_DISC_TYPE;
    PID_PARAM.DER_DISC_TYPE = CONTROL.PARAM.PITCH_ANG_PID.DER_DISC_TYPE;
    PID_PARAM.DER_INPUT = CONTROL.PARAM.PITCH_ANG_PID.DER_INPUT;
    PID_PARAM.ANTIWINDUP = CONTROL.PARAM.PITCH_ANG_PID.ANTIWINDUP;
    % PID CONTROL
    PID_OUTPUT = PID_MV(PID_INPUT,PID_PARAM);
    % OUTPUTS
    PA_MV_PRV = [PID_OUTPUT.MV PA_MV_PRV(1:end-1)];
    MOTOR_VOLT_CD(1) = PID_OUTPUT.MV;
    PA_REF_PRV = CONTROL.TARGET.PITCH_ANG_REF;
    PA_MO_PRV = CONTROL.INPUT.PITCH_ANG;
    PA_MOD_PRV = CONTROL.INPUT.PITCH_RATE;
    PA_INT_PID_PRV = PID_OUTPUT.INT;
    PA_DER_PID_PRV = PID_OUTPUT.DER;
end

%-------------------------------------------------------------------------
% FORWARD VELOCITY: DEAD BEAT
%-------------------------------------------------------------------------
if VEHICLE_MODE==0 && CONTROL_MODE>0 && CONTROL_MODE<8 && ...
        CONTROL.STATE.FORWARD_VEL_CONTROL_TYPE>=2  
    % INPUTS
    FV_DB_ERR = [CONTROL.TARGET.FORWARD_VEL_REF-CONTROL.INPUT.FORWARD_VEL FV_DB_ERR_PRV];
    FV_DB_MV = CONTROL.PARAM.FORWARD_VEL_DB.NUM*FV_DB_ERR(:) - ...
               CONTROL.PARAM.FORWARD_VEL_DB.DEN*FV_DB_MV_PRV(:);
    FV_DB_MV_PRV = [FV_DB_MV FV_DB_MV_PRV(1:end-1)];
    MOTOR_VOLT_CD(1) = FV_DB_MV;
    FV_DB_ERR_PRV = [CONTROL.TARGET.FORWARD_VEL_REF-CONTROL.INPUT.FORWARD_VEL FV_DB_ERR_PRV(1:end-1)];
end

%-------------------------------------------------------------------------
% YAW_RATE: DEAD BEAT
%-------------------------------------------------------------------------
if VEHICLE_MODE==0 && CONTROL_MODE>0 && CONTROL_MODE<8 && ...
        CONTROL.STATE.YAW_RATE_CONTROL_TYPE>=2  
    % INPUTS
    YR_DB_ERR = [CONTROL.TARGET.YAW_RATE_REF-CONTROL.INPUT.YAW_RATE YR_DB_ERR_PRV];
    YR_DB_MV = CONTROL.PARAM.YAW_RATE_DB.NUM*YR_DB_ERR(:) - ...
               CONTROL.PARAM.YAW_RATE_DB.DEN*YR_DB_MV_PRV(:);
    YR_DB_MV_PRV = [YR_DB_MV YR_DB_MV_PRV(1:end-1)];
    MOTOR_VOLT_CD(2) = YR_DB_MV;
    YR_DB_ERR_PRV = [CONTROL.TARGET.YAW_RATE_REF-CONTROL.INPUT.YAW_RATE YR_DB_ERR_PRV(1:end-1)];
end

%-------------------------------------------------------------------------
% OPEN LOOP
%-------------------------------------------------------------------------
if CONTROL_MODE==0 
    MOTOR_VOLT_CD = CONTROL.TARGET.MOTOR_VOLT_CD_REF;
end

%-------------------------------------------------------------------------
% MOTOR VOLTAGES
%-------------------------------------------------------------------------
MOTOR_VOLT_MAX = CONTROL.INPUT.BATTERY_VOLT*ones(2,1);
% MOTOR_VOLT_MAX = CONTROL.PARAM.MOTOR_VOLT_MAX;
MOTOR_VOLT = [sum(MOTOR_VOLT_CD) ; -diff(MOTOR_VOLT_CD)];
if NAV_TARGET_REACHED
    MOTOR_VOLT = zeros(2,1);
end
% DEAD ZONE
DEAD_ZONE = CONTROL.PARAM.MOTOR_DEAD_ZONE;
PWM_SLOPE = CONTROL.PARAM.MOTOR_PWM_SLOPE;
aux = [DEAD_ZONE(1)-2*PWM_SLOPE(1) DEAD_ZONE(2)+2*PWM_SLOPE(2)]';
MOTOR_VOLT = double(MOTOR_VOLT<=aux(1) | MOTOR_VOLT>=aux(2)).*MOTOR_VOLT;
% LIMITS
MOTOR_VOLT = LIMIT_MOTOR_VOLT(MOTOR_VOLT,MOTOR_VOLT_MAX);
% MOTOR_VOLT = MOTOR_VOLT.*(abs(MOTOR_VOLT)<MOTOR_VOLT_MAX) + ...
%              MOTOR_VOLT_MAX.*sign(MOTOR_VOLT).*(abs(MOTOR_VOLT)>=MOTOR_VOLT_MAX);
MOTOR_VOLT_CD = [sum(MOTOR_VOLT)/2 ; -diff(MOTOR_VOLT)/2];
% CONTROL.OUTPUT.MOTOR_VOLT_CD = [sum(MOTOR_VOLT)/2 ; -diff(MOTOR_VOLT)/2];
% CONTROL.OUTPUT.MOTOR_VOLT = MOTOR_VOLT;

end

function u_sat = LIMIT_MOTOR_VOLT(u,u_max)

u_sat = zeros(2,1);
if abs(u(1))>=abs(u(2))
    u_lim = [1 ; abs(u(2)/u(1))];
else
    u_lim = [abs(u(1)/u(2)) ; 1];
end
if abs(u(1))>=u_max(1) && abs(u(2))<u_max(2)
    u_sat(1) = sign(u(1))*u_max(1);
    u_sat(2) = u_lim(2)*u(2);
elseif abs(u(2))>=u_max(2) && abs(u(1))<u_max(1)
    u_sat(1) = u_lim(1)*u(1);
    u_sat(2) = sign(u(2))*u_max(2);
elseif abs(u(1))>=u_max(1) && abs(u(2))>=u_max(2)
    u_sat(1) = u_lim(1)*sign(u(1))*u_max(1);
    u_sat(2) = u_lim(2)*sign(u(2))*u_max(2);
else
    u_sat(1) = u(1);
    u_sat(2) = u(2);
end
end

== matlab function TEST_TCP/CONTROL/LOCAL TARGETS/WFL TARGETS/ PULSE GENERATION ==
  data: CONTROL input Bus: CONTROL_Bus; WALL_DIST_REF output
function WALL_DIST_REF = PULSE_GEN(CONTROL)
    
persistent TIMER initialize
if isempty(initialize)
    TIMER = 0;
    initialize = 1;
end

% SAMPLING TIME
SAMPLING_TIME = CONTROL.PARAM.SAMPLING_TIME; % s

%% OPERATION MODE
% / 0. BOOTING   / 1. SENSOR CALIBRATION / 2. READY
% / 3. OPEN LOOP / 4. ATTITUDE / 5. VELOCITY / 6. NAVIGATION / 
% / 7. WALL FOLLOWER / 8. WALL-FOLLOWER COMPETITION / 
% / 9. NAVIGATION COMPETITION / 10. STOP
CURRENT_STATUS = CONTROL.STATE.CURRENT_STATUS_SYS;
PREVIOUS_STATUS = CONTROL.STATE.PREVIOUS_STATUS;

if (CURRENT_STATUS == 7) && (PREVIOUS_STATUS == 7)   
    if TIMER > 15
        WALL_DIST_REF = 0.1;
    elseif TIMER < 5
        WALL_DIST_REF = 0.1;
        TIMER = TIMER + SAMPLING_TIME;
    else % 5 <= TIMER <= 15
        WALL_DIST_REF = 0.125;
        TIMER = TIMER + SAMPLING_TIME;
    end
else
    WALL_DIST_REF = 0.1;
    TIMER = 0;
end

== matlab function TEST_TCP/CONTROL/SYSTEM IDENTIFICATION/Second-order equation ==
  data: b input; r1 output; c input; r2 output
function [r1,r2] = sol_2ord_eq(b,c)
r1 = (-b+sqrt(abs(b^2-4*c)))/2;
r2 = (-b-sqrt(abs(b^2-4*c)))/2;
return

== matlab function TEST_TCP/SIMULATION/READ IMU/IMU CALIBRATION ==
  data: CONTROL_IN input; ACCEL input; ACCEL_FILT input; ACCEL_MEAN input; ACCEL_MEAN_FILT input; GYRO input; GYRO_FILT input; GYRO_MEAN input; GYRO_MEAN_FILT input; ACCEL_CALIB input; ALFA_CALIB input; ACCEL_OFFS_IN input; GYRO_OFFS_IN input; CONTROL output Bus: CONTROL_Bus; ACCEL_OFFS_OUT output; GYRO_OFFS_OUT output; GRAVITY_VECTOR input
function [CONTROL,ACCEL_OFFS_OUT,GYRO_OFFS_OUT] = IMU_CALIBRATION(CONTROL_IN,...
                       ACCEL,ACCEL_FILT,ACCEL_MEAN,ACCEL_MEAN_FILT,...
                       GYRO,GYRO_FILT,GYRO_MEAN,GYRO_MEAN_FILT,...
                       ACCEL_CALIB,ALFA_CALIB,ACCEL_OFFS_IN,GYRO_OFFS_IN,GRAVITY_VECTOR)
                        
%--------------------------------------------------------------
% COPY CONTROL BUS
%--------------------------------------------------------------
CONTROL = CONTROL_IN;

%--------------------------------------------------------------
% IMU ORIENTATION
%--------------------------------------------------------------
% ACCEL = [1 0 0 ; 0 1 0 ; 0 0 1]*ACCEL;
% GYRO = [1 0 0 ; 0 1 0 ; 0 0 1]*GYRO;
ACCEL_MEAN = [1 0 0 ; 0 1 0 ; 0 0 1]*ACCEL_MEAN;
GYRO_MEAN = [1 0 0 ; 0 1 0 ; 0 0 1]*GYRO_MEAN;
% ACCEL_FILT = [1 0 0 ; 0 1 0 ; 0 0 1]*ACCEL_FILT;
% GYRO_FILT = [1 0 0 ; 0 1 0 ; 0 0 1]*GYRO_FILT;
ACCEL_MEAN_FILT = [1 0 0 ; 0 1 0 ; 0 0 1]*ACCEL_MEAN_FILT;
GYRO_MEAN_FILT = [1 0 0 ; 0 1 0 ; 0 0 1]*GYRO_MEAN_FILT;

%--------------------------------------------------------------
% CALIBRATION 
%--------------------------------------------------------------
if CONTROL.STATE.CURRENT_STATUS_SYS == 1  % CALIBRATION ENABLED
    if ACCEL_CALIB % ACCELEROMETER CALIBRATION ENABLED
        ACCEL_OFFS_OUT = ALFA_CALIB*ACCEL_OFFS_IN + (1-ALFA_CALIB)*(ACCEL_MEAN_FILT-GRAVITY_VECTOR);
    else
        ACCEL_OFFS_OUT = ACCEL_OFFS_IN;
    end
    GYRO_OFFS_OUT  = ALFA_CALIB*GYRO_OFFS_IN  + (1-ALFA_CALIB)*GYRO_MEAN_FILT;
else % END OF CALIBRATION
    if CONTROL.STATE.VEHICLE_MODE == 1
        ACCEL_OFFS_OUT = zeros(3,1);
    else
        ACCEL_OFFS_OUT = ACCEL_OFFS_IN;
    end   
    GYRO_OFFS_OUT  = GYRO_OFFS_IN;
    % ACCEL = ACCEL - ACCEL_OFFS_OUT;
    % GYRO = GYRO - GYRO_OFFS_OUT;
    ACCEL_MEAN = ACCEL_MEAN - ACCEL_OFFS_OUT;
    GYRO_MEAN = GYRO_MEAN - GYRO_OFFS_OUT;
    % ACCEL_FILT = ACCEL_FILT - ACCEL_OFFS_OUT;
    % GYRO_FILT = GYRO_FILT - GYRO_OFFS_OUT;
    ACCEL_MEAN_FILT = ACCEL_MEAN_FILT - ACCEL_OFFS_OUT;
    GYRO_MEAN_FILT = GYRO_MEAN_FILT - GYRO_OFFS_OUT;
end

%--------------------------------------------------------------
% IMU BUS UPDATE
%--------------------------------------------------------------
CONTROL.INPUT.IMU_ACCEL_MEAN = ACCEL_MEAN;
CONTROL.INPUT.IMU_GYRO_MEAN = GYRO_MEAN;
CONTROL.INPUT.IMU_ACCEL_MEAN_FILT = ACCEL_MEAN_FILT;
CONTROL.INPUT.IMU_GYRO_MEAN_FILT = GYRO_MEAN_FILT;

return
